simulink model "engine"  (R2025b)
settings: Solver=VariableStepAuto  StartTime=0.0  StopTime=10.0  MaxStep=1e-4  RelTol=1e-3
values from neighbouring files (symbols this model uses):
  C_M = 1.3    [constants.m]
  C_omega = 3.15    [constants.m]
  J_dv = 7e-6    (= 7e-06)    [constants.m]
  L = L_a+L_OB    (= 0.0145)    [constants.m]
  L_OB = 0.013    [constants.m]
  R_a = 8    [constants.m]
settings Model: Creator=vladi  LastModifiedBy=vladi

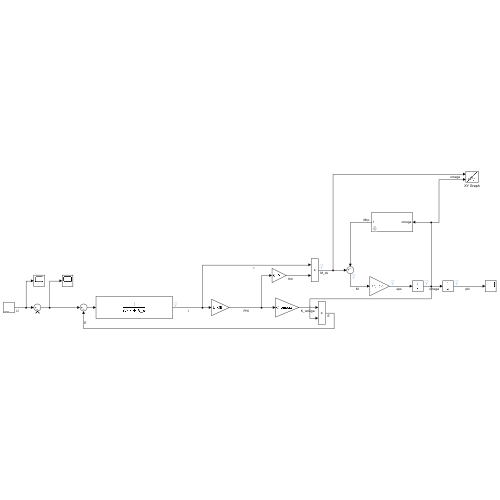
[thumbnail: Simulink's stored preview of the top-level diagram]
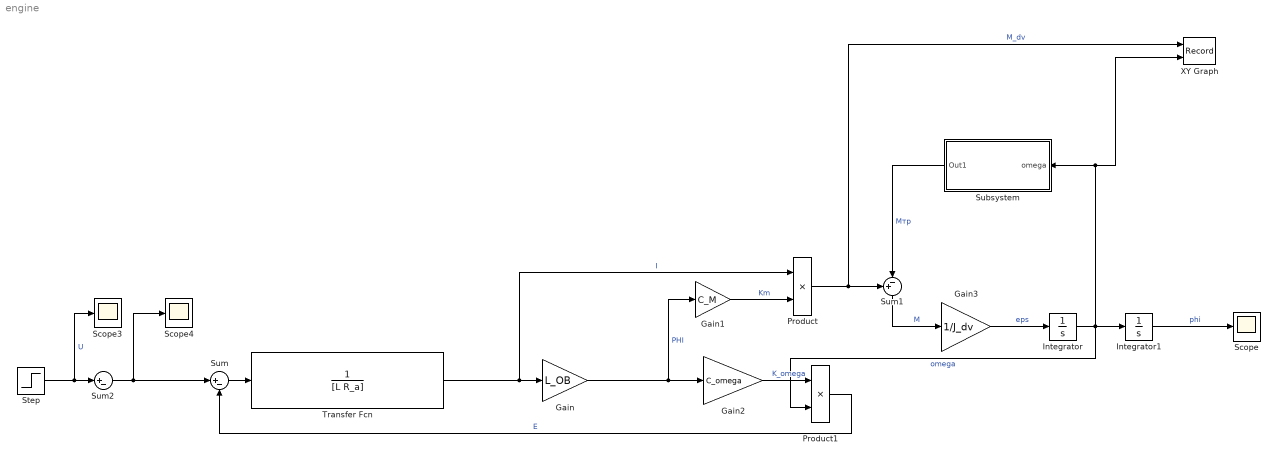
== system engine ==
  Gain : Gain  Gain=L_OB
  Gain1 : Gain  Gain=C_M
  Gain2 : Gain  Gain=C_omega
  Gain3 : Gain  Gain=1/J_dv
  Integrator : Integrator
  Integrator1 : Integrator
  Product : Product
  Product1 : Product
  Scope : Scope
      settings: ActiveDisplayYMinimum=-24.099835261611624  ActiveDisplayYMaximum=216.89851735450469
  Scope3 : Scope
      settings: ActiveDisplayYMinimum=-1  ActiveDisplayYMaximum=1  DataLoggingVariableName=ScopeData3
  Scope4 : Scope
      settings: ActiveDisplayYMinimum=-3.1249999999999991  ActiveDisplayYMaximum=28.125  DataLoggingVariableName=ScopeData4
  Step : Step  After=10  SampleTime=0
  Subsystem : Subsystem  mask{beta=1e-3}
      mask prompts: beta "Коэффициент вязкого трения"
  Sum : Sum  Inputs=|+-
  Sum1 : Sum  Inputs=+-|
  Sum2 : Sum  Inputs=|+-
  Transfer Fcn : TransferFcn  Denominator=[L R_a]
  XY Graph : Record  NumPorts=2.0  FileSettingsInternal="{\"entries\":[{\"content\":{\"excelSettings\":{\"content\":{},\"type\":\"Streamout.ExcelSettings\"},\"parquetSettings\":{\"content\":{},\"type\":\"Streamout.ParquetSettings\"}},\"type\":\"Streamout.FileSettingStorage\",\"uuid\":\"\"}],\"packageUris\":[\"http:\\/\\/schema.mathworks.com\\/mf0\\/streamout_blocks\\/R2020a\"],\"version\":\"1.0\"}"  FrameSettings=[0, 0]  Layout=[1 1]  SignalsInternal="{\"entries\":[{\"content\":{\"signals\":[{\"content\":{\"blockPath\":[],\"dimensions\":[1],\"domain\":\"\",\"lineColor\":\"#a2142f\",\"plots\":[ 1 ],\"port\":1,\"sid\":[\"\"],\"signalID\":1,\"signalName\":\"M_dv\"},\"type\":\"RecordBlkView.Signal\",\"uuid\":\"\"},{\"content\":{\"blockPath\":[],\"dimensions\":[1],\"domain\":\"\",\"lineColor\":\"#139fff\",\"plots\":[ 1 ],\"port\":2,\"sid\":[\"\"],\"signalID\":2,\"signalName\":\"omega\"},\"type\":\"RecordBlkView.Signal\",\"uuid\":\"\"}]},\"type\":\"RecordBlkView.InputSignals\",\"uuid\":\"\"}],\"packageUris\":[\"http:\\/\\/schema.mathworks.com\\/mf0\\/streamout_blocks\\/R2020a\"],\"version\":\"1.0\"}"  VisualizationBindings="{\"xyplotplugin\":{\"info\":[{\"series\":[{\"bindingParametersList\":[{\"parameter\":\"X-Axis\",\"signalID\":1,\"signalName\":\"M_dv\"},{\"parameter\":\"Y-Axis\",\"signalID\":2,\"signalName\":\"omega\"}],\"seriesID\":0}],\"subplotID\":1}]}}"  CompatibilityTag=XY
  wires:
  Gain3/1 -> Integrator/1  "eps"
  Integrator/1 -> XY Graph/2, Subsystem/1(omega), Product1/2, Integrator1/1  "omega"
  Product/1 -> XY Graph/1, Sum1/1  "M_dv"
  Product1/1 -> Sum/2  "E"
  Integrator1/1 -> Scope/1  "phi"
  Sum1/1 -> Gain3/1  "M"
  Gain2/1 -> Product1/1  "K_omega"
  Sum/1 -> Transfer Fcn/1
  Sum2/1 -> Scope4/1, Sum/1
  Gain1/1 -> Product/2  "Km"
  Transfer Fcn/1 -> Product/1, Gain/1  "I"
  Step/1 -> Scope3/1, Sum2/1  "U"
  Gain/1 -> Gain1/1, Gain2/1  "PHI"
  Subsystem/1(Out1) -> Sum1/2  "Мтр"

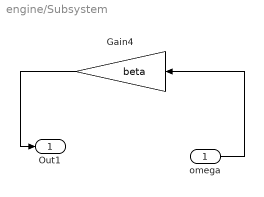
== system engine/Subsystem ==
  omega : Inport
  Gain4 : Gain  Gain=beta
  Out1 : Outport
  wires:
  Gain4/1 -> Out1/1
  omega/1 -> Gain4/1
